simulink model "EEE_316_Project_B1_Group1_final"  (R2021b)
settings: Solver=VariableStepAuto  StartTime=0.0  StopTime=5  RelTol=1e-3
values from neighbouring files (symbols this model uses):
  in1 = [1 1 0 0 0 0 0 1]    [Inputs_for_EEE316_Project.m]
  in2 = [0 0 0 1 1 1 0 0]    [Inputs_for_EEE316_Project.m]
  in3 = [0 1 1 1 0 0 0 0]    [Inputs_for_EEE316_Project.m]
  in4 = [0 0 0 0 0 1 1 1]    [Inputs_for_EEE316_Project.m]
libraries: spsIdealSwitchLib x8, simulink x4, spsSeriesRLCBranchLib x4, spsVoltageMeasurementLib x4, spsFullBridgeMMCExternalDCLinksLib x2, spsOffDelayLib x2, spsPWMGeneratorMultilevelLib x2, spsDCVoltageSourceLib x1, spsMeanLib x1, spsStepperMotorLib x1, spspowerguiLib x1
settings Model: Creator=Majumder  LastModifiedBy=Awsaf
settings SolverCC: ZeroCrossAlgorithm=Adaptive  AlgebraicLoopSolver=TrustRegion
settings DebuggingCC: IgnoredZcDiagnostic=none
settings SFSimCC: CustomCodeUndefinedFunction=UseInterfaceOnly

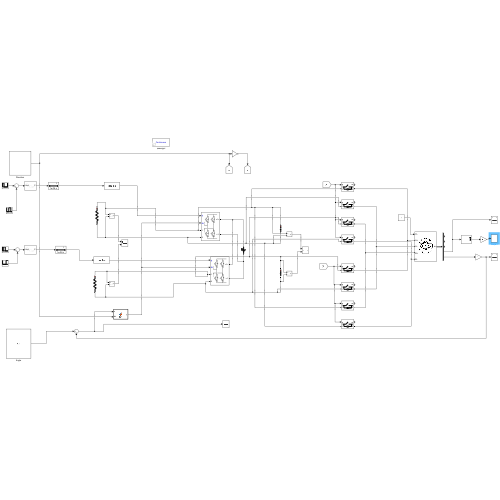
[thumbnail: Simulink's stored preview of the top-level diagram]
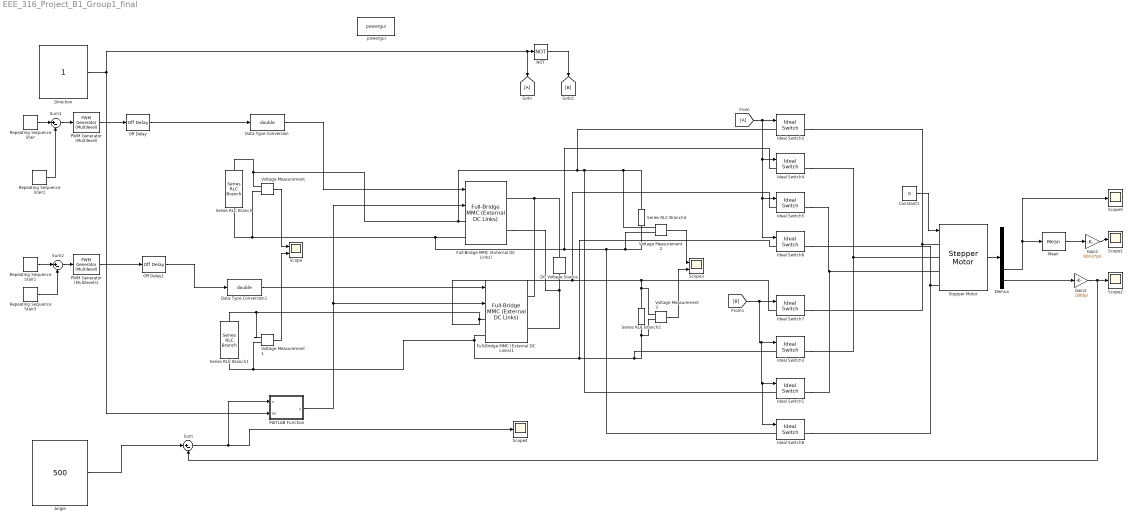
== system EEE_316_Project_B1_Group1_final ==
  Angle : Constant  Value=500
  Constant1 : Constant  Value=0
  DC Voltage Source : spsDCVoltageSourceLib/DC Voltage Source  Amplitude=20  Measurements=None
  Data Type Conversion : DataTypeConversion  OutDataTypeStr=double
  Data Type Conversion1 : DataTypeConversion  OutDataTypeStr=double
  Demux : Demux  Outputs=5
  Direction : Constant
  Full-Bridge MMC (External DC Links) : spsFullBridgeMMCExternalDCLinksLib/Full-Bridge MMC (External DC Links)  ModelType=Switching devices  n=1  Ron=1e-3  Rs=1e6  Cs=inf  Ron_Diode=1e-3  Rs_Diode=1e6  Cs_Diode=inf  Vf_Diode=1e-3  Rs_CurrentSource=inf  Ts=10e-6
      settings: SourceProductBaseCode=PS
  Full-Bridge MMC (External DC Links)1 : spsFullBridgeMMCExternalDCLinksLib/Full-Bridge MMC (External DC Links)  ModelType=Switching devices  n=1  Ron=1e-3  Rs=1e6  Cs=inf  Ron_Diode=1e-3  Rs_Diode=1e6  Cs_Diode=inf  Vf_Diode=1e-3  Rs_CurrentSource=inf  Ts=10e-6
      settings: SourceProductBaseCode=PS
  Gain1 : Gain  Gain=60/(2*pi)
  Gain2 : Gain  Gain=180/pi
  Ideal Switch{1..8} (8 alike) : spsIdealSwitchLib/Ideal Switch  Ron=0.001  Lon=0  IC=0  Rs=1e5  Cs=inf  Measurements=on
  MATLAB Function : MATLAB Function  TreatAsAtomicUnit=on
  Mean : spsMeanLib/Mean  Freq=f  Vinit=0  Ts=0
  NOT : Logic  Operator=NOT  IconShape=distinctive  AllPortsSameDT=off  OutDataTypeStr=boolean
  Off Delay : spsOffDelayLib/Off Delay  DelayType=Off delay  delay=1e-6  ic=1  Ts=0
      settings: SourceProductBaseCode=PS
  Off Delay1 : spsOffDelayLib/Off Delay  DelayType=Off delay  delay=1e-6  ic=1  Ts=0
      settings: SourceProductBaseCode=PS
  PWM Generator (Multilevel) : spsPWMGeneratorMultilevelLib/PWM Generator (Multilevel)  BridgeType=Full-bridge  NumberOfBridges=1  Fc=540  Ts=0  ShowCarriersOutport=off
      settings: SourceProductBaseCode=PS
  PWM Generator (Multilevel)1 : spsPWMGeneratorMultilevelLib/PWM Generator (Multilevel)  BridgeType=Full-bridge  NumberOfBridges=1  Fc=540  Ts=0  ShowCarriersOutport=off
      settings: SourceProductBaseCode=PS
  Repeating Sequence Stair : simulink/Sources/Repeating Sequence Stair  OutValues=in1.'  tsamp=S  OutMin=[]  OutMax=[]  OutDataTypeStr=double  OutputDataTypeScalingMode=double  OutDataType=fixdt(0,8)  ConRadixGroup=Best Precision: Vector-wise  OutScaling=2^-12
  Repeating Sequence Stair1 : simulink/Sources/Repeating Sequence Stair  OutValues=in3.'  tsamp=S  OutMin=[]  OutMax=[]  OutDataTypeStr=double  OutputDataTypeScalingMode=double  OutDataType=fixdt(0,8)  ConRadixGroup=Best Precision: Vector-wise  OutScaling=2^-12
  Repeating Sequence Stair2 : simulink/Sources/Repeating Sequence Stair  OutValues=in2.'  tsamp=S  OutMin=[]  OutMax=[]  OutDataTypeStr=double  OutputDataTypeScalingMode=double  OutDataType=fixdt(0,8)  ConRadixGroup=Best Precision: Vector-wise  OutScaling=2^-12
  Repeating Sequence Stair3 : simulink/Sources/Repeating Sequence Stair  OutValues=in4.'  tsamp=S  OutMin=[]  OutMax=[]  OutDataTypeStr=double  OutputDataTypeScalingMode=double  OutDataType=fixdt(0,8)  ConRadixGroup=Best Precision: Vector-wise  OutScaling=2^-12
  Scope : Scope  NumInputPorts=2
  Scope{1..2,4..5} (4 alike) : Scope
  Scope3 : Scope  NumInputPorts=2
  Series RLC Branch : spsSeriesRLCBranchLib/Series RLC Branch  LConnTagsString=__new0  RConnTagsString=__new0  BranchType=R  Resistance=1000  Inductance=0  SetiL0=off  InitialCurrent=0  Capacitance=0  Setx0=off  InitialVoltage=0  Measurements=None
  Series RLC Branch1 : spsSeriesRLCBranchLib/Series RLC Branch  LConnTagsString=__new0  RConnTagsString=__new0  BranchType=R  Resistance=1000  Inductance=0  SetiL0=off  InitialCurrent=0  Capacitance=0  Setx0=off  InitialVoltage=0  Measurements=None
  Series RLC Branch2 : spsSeriesRLCBranchLib/Series RLC Branch  LConnTagsString=__new0  RConnTagsString=__new0  BranchType=C  Resistance=1  Inductance=1e-3  SetiL0=off  InitialCurrent=0  Capacitance=1e-7  Setx0=off  InitialVoltage=0  Measurements=None
  Series RLC Branch4 : spsSeriesRLCBranchLib/Series RLC Branch  LConnTagsString=__new0  RConnTagsString=__new0  BranchType=C  Resistance=1  Inductance=1e-3  SetiL0=off  InitialCurrent=0  Capacitance=1e-7  Setx0=off  InitialVoltage=0  Measurements=None
  Stepper Motor : spsStepperMotorLib/Stepper Motor  MotorType=Permanent-magnet / Hybrid  NumberOfPhases_1=2  NumberOfPhases_2=3  PresetModel_1=<empty>  PresetModel_2=<empty>  L=10e-3  Lmax=10e-3  Lmin=2e-3  R=1.2  Step_angle=1.8  Psim=0.04  Tdm=0.02  J=1e-4/5  B=1e-3  w0=0  pos0=0  TsPowergui=0  TsBlock=-1
      settings: SourceProductBaseCode=PS
  Sum : Sum  Inputs=|+-
  Sum1 : Sum  Inputs=|+-
  Sum2 : Sum  Inputs=|+-
  Voltage Measurement{,1..3} (4 alike) : spsVoltageMeasurementLib/Voltage Measurement  PhasorSimulation=off  OutputType=Complex  PSBequivalent=0
  powergui : spspowerguiLib/powergui  Priority=1  SimulationMode=Continuous  SampleTime=50e-6  frequency=60  Iterations=50  frequencyindice=0  Pbase=100e6  ErrMax=1e-4  UnitsV=kV  UnitsW=MW  buscounter=0  FunctionMessages=off  echomessages=off  EnableUseOfTLC=off  CurrentSourceSwitches=off  DisableSnubberDevices=off  DisableRonSwitches=off  DisableVfSwitches=off  DisplayEquations=off  AutomaticDiscreteSolvers=off  SolverType=Tustin/Backward Euler (TBE)  Interpol=off  ExternalGateDelay=off  methode=off  Ts=100  x0status=blocks  SPID=on  SwTol=0  HookPort=off  NonlinearTolerance=1e-4  nMaxIteration=100  ContinueOnMaxIteration=off  RestoreLinks=warning  ResistiveCurrentMeasurement=off  Frange=[0:2:500]  Ylog=off  Xlog=on  ShowGrid=off  save=off  variable=ZData  structure=0  ZoomFFT=off  StartTime=0.0  cycles=1  DisplayStyle=1  fundamental=60  FreqAxis=off  MaxFrequency=1000  frequencyindicesteady=1  RmsSteady=1  display=off
  wires:
  Voltage Measurement/1 -> Scope/1
  Stepper Motor/1 -> Demux/1
  Gain1/1 -> Scope1/1
  Demux/5 -> Gain2/1
  Gain2/1 -> Sum/2, Scope2/1
  Constant1/1 -> Stepper Motor/1
  Demux/4 -> Scope5/1, Mean/1
  Mean/1 -> Gain1/1
  Direction/1 -> [A], NOT/1, MATLAB Function/2(dir)
  NOT/1 -> [B]
  [A] -> Ideal Switch6/1, Ideal Switch5/1, Ideal Switch4/1, Ideal Switch2/1
  [B] -> Ideal Switch8/1, Ideal Switch1/1, Ideal Switch3/1, Ideal Switch7/1
  Voltage Measurement2/1 -> Scope3/1
  Voltage Measurement3/1 -> Scope3/2
  Angle/1 -> Sum/1
  Voltage Measurement1/1 -> Scope/2
  Sum/1 -> MATLAB Function/1(u), Scope4/1
  MATLAB Function/1(y) -> Full-Bridge MMC (External DC Links)1/2, Full-Bridge MMC (External DC Links)/2
  Repeating Sequence Stair/1 -> Sum1/1
  Sum1/1 -> PWM Generator (Multilevel)/1
  Repeating Sequence Stair2/1 -> Sum1/2
  Repeating Sequence Stair1/1 -> Sum2/1
  Repeating Sequence Stair3/1 -> Sum2/2
  Sum2/1 -> PWM Generator (Multilevel)1/1
  PWM Generator (Multilevel)1/1 -> Off Delay1/1
  PWM Generator (Multilevel)/1 -> Off Delay/1
  Off Delay/1 -> Data Type Conversion/1
  Data Type Conversion/1 -> Full-Bridge MMC (External DC Links)/1
  Data Type Conversion1/1 -> Full-Bridge MMC (External DC Links)1/1
  Off Delay1/1 -> Data Type Conversion1/1
  connections:
  DC Voltage Source/RConn1 -- Full-Bridge MMC (External DC Links)1/RConn1 -- Full-Bridge MMC (External DC Links)/RConn1
  DC Voltage Source/LConn1 -- Full-Bridge MMC (External DC Links)/RConn2 -- Full-Bridge MMC (External DC Links)1/RConn2
  Full-Bridge MMC (External DC Links)/LConn2 -- Ideal Switch8/LConn1 -- Voltage Measurement2/LConn2 -- Series RLC Branch4/RConn1 -- Ideal Switch4/LConn1 -- Voltage Measurement/LConn2 -- Series RLC Branch/RConn1
  Full-Bridge MMC (External DC Links)/LConn1 -- Ideal Switch1/LConn1 -- Voltage Measurement2/LConn1 -- Series RLC Branch4/LConn1 -- Ideal Switch2/LConn1 -- Voltage Measurement/LConn1 -- Series RLC Branch/LConn1
  Full-Bridge MMC (External DC Links)1/LConn1 -- Voltage Measurement3/LConn1 -- Series RLC Branch2/LConn1 -- Ideal Switch7/LConn1 -- Ideal Switch5/LConn1 -- Voltage Measurement1/LConn1 -- Series RLC Branch1/LConn1
  Full-Bridge MMC (External DC Links)1/LConn2 -- Voltage Measurement3/LConn2 -- Series RLC Branch2/RConn1 -- Ideal Switch3/LConn1 -- Ideal Switch6/LConn1 -- Voltage Measurement1/LConn2 -- Series RLC Branch1/RConn1
  Ideal Switch2/RConn1 -- Ideal Switch7/RConn1 -- Stepper Motor/LConn1
  Ideal Switch4/RConn1 -- Ideal Switch3/RConn1 -- Stepper Motor/LConn2
  Ideal Switch5/RConn1 -- Ideal Switch1/RConn1 -- Stepper Motor/LConn3
  Ideal Switch8/RConn1 -- Ideal Switch6/RConn1 -- Stepper Motor/LConn4

== matlab function EEE_316_Project_B1_Group1_final/MATLAB Function ==
  data: u input; y output; dir input
function y  = fcn(u,dir)
    if dir == 1
        if (u < 0)
            y = 1;
        else
            y = 0;
        end
    elseif dir == 0
            if (u> 0)
                y = 1;
            else
                y = 0;
            end
    else
        y = 0;
    end
end
